simulink model "VariableCylinderTest"  (R2017b)
settings: Solver=ode15s  StartTime=0.0  StopTime=5  RelTol=1e-3  EnableMultiTasking=on
undefined symbols (not defined in the file): spring1kd, spring1ks, teth_length, teth_numLinks, teth_radius, X, Y, Z
libraries: sm_lib x16, nesl_utility x11, SimMainLibrary x5, vrlib x2, simulink x1, powerlib_meascontrol x1
settings Model: Creator=Aaron  LastModifiedBy=Aaron
settings DataIOCC: LimitDataPoints=on
settings OptimizationCC: LifeSpan=inf
settings DebuggingCC: AllowSymbolicDim=off  SFUnexpectedBacktrackingDiag=warning  SFNoUnconditionalDefaultTransitionDiag=warning  SFExecutionAtInitializationDiag=none
settings CodeAppCC: StateflowObjectComments=on
settings GRTTargetCC: TargetLangStandard=C89/C90 (ANSI)  GeneratePreprocessorConditionals=Disable all
settings ConfigComp: CovMetricSettings=dw  CovHtmlReporting=on  CovSaveCumulativeToWorkspaceVar=on  CovSaveSingleToWorkspaceVar=on  CovExternalEMLEnable=off  CovSFcnEnable=off
settings SimscapeCC: SimscapeNominalValues="[{\"value\":\"10\",\"unit\":\"V\"},{\"value\":\"1\",\"unit\":\"A\"},{\"value\":\"10\",\"unit\":\"N*m\"},{\"value\":\"10\",\"unit\":\"bar\"},{\"value\":\"100\",\"unit\":\"kJ/kg\"},{\"value\":\"1\",\"unit\":\"kW\"},{\"value\":\"300\",\"unit\":\"K\"},{\"value\":\"100\",\"unit\":\"cm^3/s\"},{\"value\":\"1\",\"unit\":\"kN\"},{\"value\":\"1\",\"unit\":\"g/cm^3\"},{\"value\":\"1\",\"unit\":\"l\"},{\"value\":\"1\",\"unit\":\"cm^2\"},{\"value\":\"60\",\"unit\":\"Hz\"}]"  SimscapeLogType=all  SimscapeLogDataHistory=10000
settings ConfigurationSet: Description=SimMechanics 2G
settings ExplorerConfigSet: InternalSimMechanicsExplorerSettings="<ExplorerConfiguration><canonicalview>default</canonicalview><AnimationSetting><BasePlaybackSpeed>1.0</BasePlaybackSpeed><PlaybackSpeedFactor>1.0</PlaybackSpeedFactor></AnimationSetting><TilePanel><TileInfo><Tiles Columns=\"1\" Count=\"1\" Rows=\"1\"><Column Weight=\"1\"/><Row Weight=\"1\"/><Tile Height=\"1\" Width=\"1\" X=\"0\" Y=\"0\"/></Tiles></TileInfo><SceneInfo><SceneViewer><BGColor><R>1</R><G>1</G><B>1</B></BGColor><Camera><DoPerspective>on</DoPerspective><Position><X>1.5</X><Y>0.241749665669615088</Y><Z>0.970338651785359607</Z></Position><Center><X>0.926423563648953952</X><Y>0.0437199328301693946</Y><Z>0.175483761522758019</Z></Center><Up><X>0.81915204428899191</X><Y>-0.138661911723834602</Y><Z>-0.556563385944725209</Z></Up><ViewLimDist>1</ViewLimDist><YLim>0.466307658154998583</YLim><XLim>1.37343348832790579</XLim></Camera></SceneViewer></SceneInfo></TilePanel><MechEditorPanel><Cameras><Camera><Id>Camera1</Id><Value><Name>Camera1</Name><NativeCamera><PositionTrackingFeature>Camera_Frame.F</PositionTrackingFeature><CenterTrackingFeature>Camera_Frame.F</CenterTrackingFeature><UpVectorTrackingFeature>Camera_Frame.F</UpVectorTrackingFeature><CenterTrackingOrigin>off</CenterTrackingOrigin><CenterTrackingDirection>-Y</CenterTrackingDirection><UpVectorTrackingDirection>+X</UpVectorTrackingDirection></NativeCamera></Value></Camera></Cameras><GfxPanelCameraMap><MapElement CameraMLId=\"Camera1\" GfxPanelIndex=\"0\"/></GfxPanelCameraMap><VideoCreator><PlaybackSpeedRatio>1.0</PlaybackSpeedRatio><FrameRate>30</FrameRate><VideoFormat>Motion JPEG AVI</VideoFormat><FrameSize>auto</FrameSize></VideoCreator></MechEditorPanel></ExplorerConfiguration>"

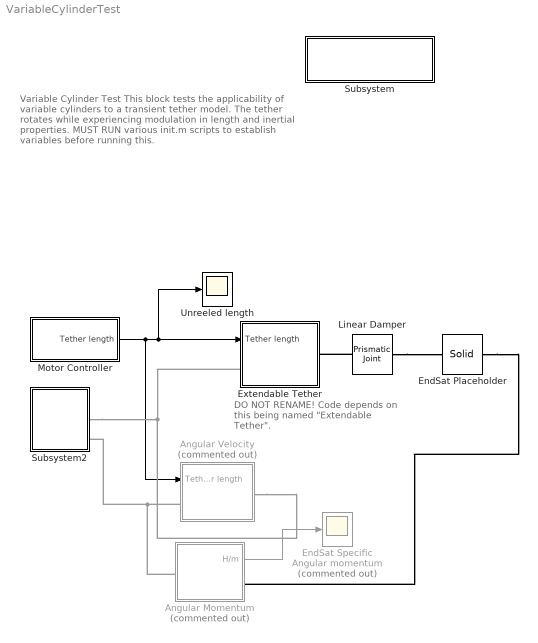
== system VariableCylinderTest ==
  note: DO NOT RENAME! Code depends on this being named "Extendable Tether".
  note: Variable Cylinder Test
      | This block tests the applicability of variable cylinders to a transient tether model. The tether rotates while experiencing modulation in length and inertial properties.
      | MUST RUN various init.m scripts to establish variables before running this.
  Angular Momentum : Subsystem  Commented=on
  Angular Velocity : Subsystem  Commented=on
  EndSat Placeholder : sm_lib/Body Elements/Solid  InertiaType=Custom  Mass=1  MassUnits=kg  CenterOfMass=[0 0 0]  CenterOfMassUnits=m  MomentsOfInertia=[.01 .01 .01]  MomentsOfInertiaUnits=kg*m^2  ProductsOfInertia=[0 0 0]  ProductsOfInertiaUnits=kg*m^2  DensityBased=off  Density=100000  DensityUnits=kg/m^3  DoExposeReferenceFrame=on  SerializedFrames=<Frames><Frame><Id>Frame1</Id><Value><Name>F1</Name><Origin><Source>GeometricFeature</Source><FeatureName>-z surface</FeatureName></Origin><PrimaryAxis><DefinedDirection>+Z</DefinedDirection><Source>ReferenceFrame</Source><SourceDirection>+Z</SourceDirection><FeatureName></FeatureName></PrimaryAxis><SecondaryAxis><DefinedDirection>+X</DefinedDirection><Source>ReferenceFrame</Source><SourceDirection>+X</SourceDirection><FeatureName></FeatureName></SecondaryAxis></Value></Frame></Frames>  GraphicType=FromGeometry  MarkerShape=Sphere  MarkerSize=10  GraphicVisPropType=SimpleVisualProperties  GraphicDiffuseColor=[0.5 0.5 0.5]  GraphicSpecularColor=[0.5 0.5 0.5 1.0]  GraphicAmbientColor=[0.15 0.15 0.15 1.0]  GraphicEmissiveColor=[0.0 0.0 0.0 1.0]  GraphicShininess=75  GraphicOpacity=1.0  GeometryShape=Brick  RectangleSize=[1 1]  RectangleSizeUnits=m  BrickDimensions=[.1 0.1 .1]  BrickDimensionUnits=m  CylinderRadius=.1  CylinderRadiusUnits=m  CylinderLength=1  CylinderLengthUnits=m  SphereRadius=1  SphereRadiusUnits=m  EllipsoidRadii=[1 1 1]  EllipsoidRadiiUnits=m  ExtrusionCrossSection=[1 1; -1 1; -1 -1; 1 -1]  ExtrusionCrossSectionUnits=m  ExtrusionLength=1  ExtrusionLengthUnits=m  PolygonNumSides=3  PolygonOuterRadius=1  PolygonOuterRadiusUnits=m  ExtGeomFileType=STEP  ExtGeomFileUnits=m  RevolutionCrossSection=[1 1; 1 -1; 2 -1; 2 1]  RevolutionCrossSectionUnits=m  RevolutionExtent=Full  RevolutionAngle=180  RevolutionAngleUnits=deg
  EndSat Specific Angular momentum : Scope  Commented=on
  Extendable Tether : Subsystem
  Linear Damper : sm_lib/Joints/Prismatic Joint  SenseConstraintForce=off  SenseConstraintForceX=off  SenseConstraintForceY=off  SenseConstraintForceZ=off  SenseConstraintTorque=off  SenseConstraintTorqueX=off  SenseConstraintTorqueY=off  SenseConstraintTorqueZ=off  SenseTotalForce=off  SenseTotalForceX=off  SenseTotalForceY=off  SenseTotalForceZ=off  SenseTotalTorque=off  SenseTotalTorqueX=off  SenseTotalTorqueY=off  SenseTotalTorqueZ=off  CompositeWrenchDir=FollowerOnBase  CompositeWrenchFrame=BaseFrame  EquilibriumPosition=0  EquilibriumPositionUnits=m  SpringStiffness=500  SpringStiffnessUnits=N/m  DampingCoefficient=50  DampingCoefficientUnits=N/(m/s)  TorqueActuationMode=NoTorque  MotionActuationMode=ComputedMotion  SensePosition=off  SenseVelocity=off  SenseAcceleration=off  SenseTorqueForce=off  PositionTargetSpecify=off  PositionTargetPriority=High  PositionTargetValue=0  PositionTargetValueUnits=m  VelocityTargetSpecify=off  VelocityTargetPriority=High  VelocityTargetValue=0  VelocityTargetValueUnits=m/s
  Motor Controller : Subsystem
  Subsystem : Subsystem
      settings: OpenFcn=open_system('sm_lib')
      mask Display: disp(sprintf('Open Simscape Multibody\nLibrary'));
  Subsystem2 : Subsystem
  Unreeled length : Scope
  wires:
  Angular Momentum/1(H/m) -> EndSat Specific Angular momentum/1
  Motor Controller/1(Tether length) -> Extendable Tether/1(Tether length), Unreeled length/1, Angular Velocity/1(Tether length)
  connections:
  EndSat Placeholder/RConn1 -- Angular Momentum/RConn1
  Linear Damper/RConn1 -- Extendable Tether/RConn1
  Linear Damper/LConn1 -- EndSat Placeholder/LConn1
  Angular Velocity/RConn1 -- Subsystem2/RConn2 -- Extendable Tether/LConn1
  Angular Velocity/LConn1 -- Subsystem2/RConn3 -- Angular Momentum/LConn1

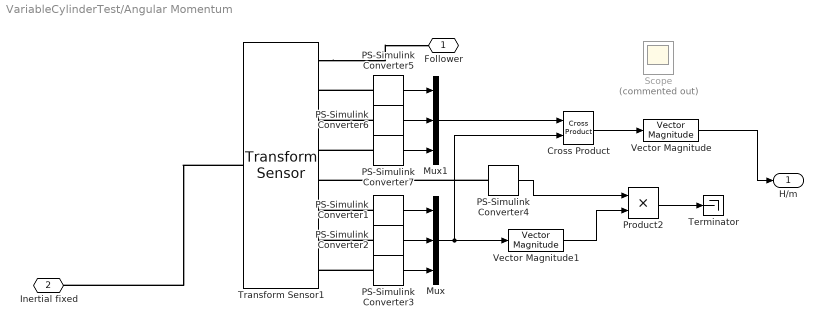
== system VariableCylinderTest/Angular Momentum ==
  Cross Product : vrlib/Utilities/Cross Product
      settings: SourceProductBaseCode=VR
  Mux : Mux  Inputs=3
  Mux1 : Mux  Inputs=3
  PS-Simulink Converter1 : nesl_utility/PS-Simulink Converter  PhysicalDomain=network_engine_domain  SubClassName=ps_output  LeftPortType=input  RightPortType=output  PseudoPeriodic=off  Frequencies=[]  Unit=m/s  AffineConversion=off
  PS-Simulink Converter2 : nesl_utility/PS-Simulink Converter  PhysicalDomain=network_engine_domain  SubClassName=ps_output  LeftPortType=input  RightPortType=output  PseudoPeriodic=off  Frequencies=[]  Unit=m/s  AffineConversion=off
  PS-Simulink Converter3 : nesl_utility/PS-Simulink Converter  PhysicalDomain=network_engine_domain  SubClassName=ps_output  LeftPortType=input  RightPortType=output  PseudoPeriodic=off  Frequencies=[]  Unit=m/s  AffineConversion=off
  PS-Simulink Converter{4..7} (4 alike) : nesl_utility/PS-Simulink Converter  PhysicalDomain=network_engine_domain  SubClassName=ps_output  LeftPortType=input  RightPortType=output  PseudoPeriodic=off  Frequencies=[]  Unit=m  AffineConversion=off
  Product2 : Product
  Scope : Scope  Commented=on  NumInputPorts=2
  Terminator : Terminator
  Transform Sensor1 : sm_lib/Frames and Transforms/Transform Sensor  MeasurementFrame=Base  SenseAngle=off  SenseAxis=off  SenseAngle1=off  SenseAngle2=off  SenseAngle3=off  SenseQ=off  SenseR=off  SenseOmegaX=off  SenseOmegaY=off  SenseOmegaZ=off  SenseOmega1=off  SenseOmega2=off  SenseOmega3=off  SenseQDot=off  SenseRDot=off  SenseAlphaX=off  SenseAlphaY=off  SenseAlphaZ=off  SenseAlpha1=off  SenseAlpha2=off  SenseAlpha3=off  SenseQDDot=off  SenseRDDot=off  SenseX=on  SenseY=on  SenseZ=on  SenseRad=off  SenseAzim=off  SenseDist=on  SenseInc=off  SenseXDot=on  SenseYDot=on  SenseZDot=on  SenseRadDot=off  SenseAzimDot=off  SenseDistDot=off  SenseIncDot=off  SenseXDDot=off  SenseYDDot=off  SenseZDDot=off  SenseRadDDot=off  SenseAzimDDot=off  SenseDistDDot=off  SenseIncDDot=off
  Vector Magnitude : SimMainLibrary/Vector Magnitude
  Vector Magnitude1 : SimMainLibrary/Vector Magnitude
  Follower : PMIOPort  Port=1  Side=Right
  Inertial fixed : PMIOPort  Port=2  Side=Left
  H/m : Outport
  wires:
  PS-Simulink Converter2/1 -> Mux/2
  PS-Simulink Converter3/1 -> Mux/3
  PS-Simulink Converter4/1 -> Product2/1
  Mux/1 -> Vector Magnitude1/1, Cross Product/2
  PS-Simulink Converter1/1 -> Mux/1
  Vector Magnitude1/1 -> Product2/2
  PS-Simulink Converter7/1 -> Mux1/3
  PS-Simulink Converter5/1 -> Mux1/1
  PS-Simulink Converter6/1 -> Mux1/2
  Mux1/1 -> Cross Product/1
  Product2/1 -> Terminator/1
  Vector Magnitude/1 -> H/m/1
  Cross Product/1 -> Vector Magnitude/1
  connections:
  PS-Simulink Converter3/LConn1 -- Transform Sensor1/RConn8
  Transform Sensor1/LConn1 -- Inertial fixed/RConn1
  Transform Sensor1/RConn1 -- Follower/RConn1
  PS-Simulink Converter2/LConn1 -- Transform Sensor1/RConn7
  PS-Simulink Converter4/LConn1 -- Transform Sensor1/RConn5
  PS-Simulink Converter1/LConn1 -- Transform Sensor1/RConn6
  PS-Simulink Converter5/LConn1 -- Transform Sensor1/RConn2
  PS-Simulink Converter6/LConn1 -- Transform Sensor1/RConn3
  PS-Simulink Converter7/LConn1 -- Transform Sensor1/RConn4

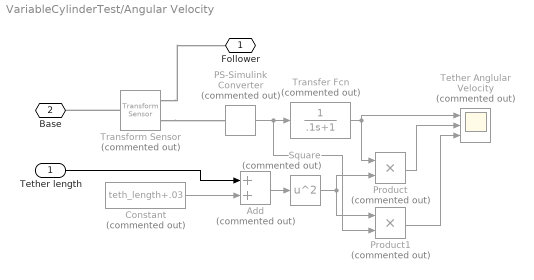
== system VariableCylinderTest/Angular Velocity ==
  Tether length : Inport
  Add : Sum  Commented=on
  Constant : Constant  Commented=on  Value=teth_length+.03
  PS-Simulink Converter : nesl_utility/PS-Simulink Converter  Commented=on  PhysicalDomain=network_engine_domain  SubClassName=ps_output  LeftPortType=input  RightPortType=output  PseudoPeriodic=off  Frequencies=[]  Unit=rad/s  AffineConversion=off
  Product : Product  Commented=on
  Product1 : Product  Commented=on
  Square : Math  Commented=on  Operator=square  RndMeth=Zero  SaturateOnIntegerOverflow=on
  Tether Anglular Velocity : Scope  Commented=on  NumInputPorts=3
  Transfer Fcn : TransferFcn  Commented=on  Denominator=[.1 1]
  Transform Sensor : sm_lib/Frames and Transforms/Transform Sensor  Commented=on  MeasurementFrame=Base  SenseAngle=off  SenseAxis=off  SenseAngle1=off  SenseAngle2=off  SenseAngle3=off  SenseQ=off  SenseR=off  SenseOmegaX=on  SenseOmegaY=off  SenseOmegaZ=off  SenseOmega1=off  SenseOmega2=off  SenseOmega3=off  SenseQDot=off  SenseRDot=off  SenseAlphaX=off  SenseAlphaY=off  SenseAlphaZ=off  SenseAlpha1=off  SenseAlpha2=off  SenseAlpha3=off  SenseQDDot=off  SenseRDDot=off  SenseX=off  SenseY=off  SenseZ=off  SenseRad=off  SenseAzim=off  SenseDist=off  SenseInc=off  SenseXDot=off  SenseYDot=off  SenseZDot=off  SenseRadDot=off  SenseAzimDot=off  SenseDistDot=off  SenseIncDot=off  SenseXDDot=off  SenseYDDot=off  SenseZDDot=off  SenseRadDDot=off  SenseAzimDDot=off  SenseDistDDot=off  SenseIncDDot=off
  Follower : PMIOPort  Port=1  Side=Right
  Base : PMIOPort  Port=2  Side=Left
  wires:
  Product1/1 -> Tether Anglular Velocity/3
  Tether length/1 -> Add/1
  Product/1 -> Tether Anglular Velocity/2
  Transfer Fcn/1 -> Product/1, Tether Anglular Velocity/1
  Add/1 -> Square/1
  Constant/1 -> Add/2
  Square/1 -> Product1/1, Product/2
  PS-Simulink Converter/1 -> Product1/2, Transfer Fcn/1
  connections:
  Transform Sensor/RConn1 -- Follower/RConn1
  Transform Sensor/LConn1 -- Base/RConn1
  Transform Sensor/RConn2 -- PS-Simulink Converter/LConn1

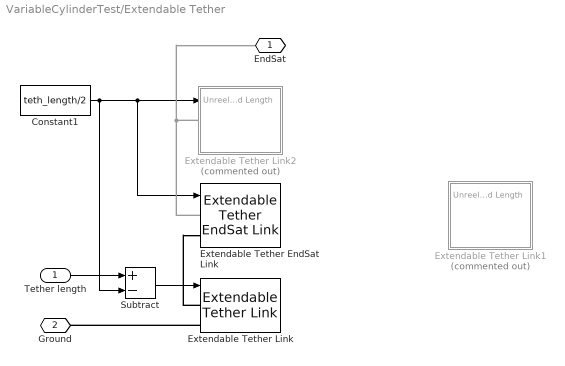
== system VariableCylinderTest/Extendable Tether ==
  Tether length : Inport
  Constant1 : Constant  Value=teth_length/2
  Extendable Tether EndSat Link : SimMainLibrary/Extendable Tether EndSat Link
  Extendable Tether Link : SimMainLibrary/Extendable Tether Link
  Extendable Tether Link1 : Subsystem  Commented=on
  Extendable Tether Link2 : Subsystem  Commented=on
  Subtract : Sum  Inputs=+-
  EndSat : PMIOPort  Port=1  Side=Right
  Ground : PMIOPort  Port=2  Side=Left
  wires:
  Constant1/1 -> Subtract/2, Extendable Tether EndSat Link/1, Extendable Tether Link2/1(Unreeled Length)
  Tether length/1 -> Subtract/1
  Subtract/1 -> Extendable Tether Link/1
  connections:
  Extendable Tether Link/LConn1 -- Extendable Tether EndSat Link/LConn2
  Extendable Tether Link/LConn2 -- Ground/RConn1
  Extendable Tether Link2/LConn1 -- Extendable Tether EndSat Link/LConn1 -- EndSat/RConn1

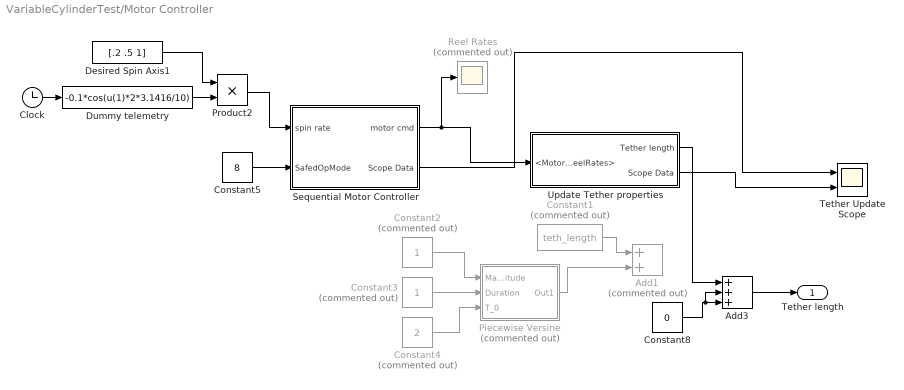
== system VariableCylinderTest/Motor Controller ==
  Add1 : Sum  Commented=on
  Add3 : Sum  Inputs=+++
  Clock : Clock
  Constant1 : Constant  Commented=on  Value=teth_length
  Constant2 : Constant  Commented=on
  Constant3 : Constant  Commented=on
  Constant4 : Constant  Commented=on  Value=2
  Constant5 : Constant  Value=8
  Constant8 : Constant  Value=0
  Desired Spin Axis1 : Constant  Value=[.2 .5 1]
  Dummy telemetry : Fcn  Expr=-0.1*cos(u(1)*2*3.1416/10)
  Piecewise Versine : Subsystem  Commented=on
  Product2 : Product
  "Reel Rates " : Scope  Commented=on
  "Sequential Motor Controller " : Subsystem  AncestorBlock=SimMainLibrary/Sequential Motor Controller
  Tether Update Scope : Scope  NumInputPorts=2
  Update Tether properties : Subsystem  AncestorBlock=SimMainLibrary/Update Tether properties
  Tether length : Outport
  wires:
  Product2/1 -> "Sequential Motor Controller "/1(spin rate)
  Constant5/1 -> "Sequential Motor Controller "/2(SafedOpMode)
  Update Tether properties/2(Scope Data) -> Tether Update Scope/2
  Constant2/1 -> Piecewise Versine/1(Magnitude)
  Piecewise Versine/1(Out1) -> Add1/2
  "Sequential Motor Controller "/1(motor cmd) -> Update Tether properties/1(<MotorReelRates>), "Reel Rates "/1
  Constant1/1 -> Add1/1
  Constant4/1 -> Piecewise Versine/3(T_0)
  Constant3/1 -> Piecewise Versine/2(Duration)
  Constant8/1 -> Add3/2, Add3/3
  Add3/1 -> Tether length/1
  Update Tether properties/1(Tether length) -> Add3/1
  Dummy telemetry/1 -> Product2/2
  Clock/1 -> Dummy telemetry/1
  Desired Spin Axis1/1 -> Product2/1
  "Sequential Motor Controller "/2(Scope Data) -> Tether Update Scope/1

== system VariableCylinderTest/Subsystem ==

== system VariableCylinderTest/Subsystem2 ==
  Camera Frame : sm_lib/Frames and Transforms/Rigid Transform  TranslationMethod=Cartesian  TranslationStandardOffset=0  TranslationLengthUnit=m  TranslationStandardAxis=+Z  TranslationCartesianOffset=[1.5 1 0]  TranslationROffset=0  TranslationROffsetUnits=m  TranslationZOffset=0  TranslationZOffsetUnits=m  TranslationThetaOffset=0  TranslationThetaOffsetUnits=deg  RotationMethod=StandardAxis  RotationAngleUnits=deg  RotationStandardAxis=+Z  RotationAngle=-35  RotationArbitraryAxis=[0 0 1]  FollAlignAxisA=+X  BaseAlignAxisA=+Y  FollAlignAxisB=+Y  BaseAlignAxisB=+Z  RotationSequenceAxes=FollowerAxes  RotationSequence=XYX  RotationSequenceAngles=[0 0 0]  RotationSequenceAnglesUnits=deg  RotationMatrix=[1 0 0; 0 1 0; 0 0 1]
  Mechanism Configuration : sm_lib/Utilities/Mechanism Configuration  UniformGravity=None  GravityVector=[0 0 -9.80665]  GravityUnits=m/s^2  LinearizationDelta=0.001
  Rigid Transform : sm_lib/Frames and Transforms/Rigid Transform  TranslationMethod=StandardAxis  TranslationStandardOffset=0  TranslationLengthUnit=m  TranslationStandardAxis=+Y  TranslationCartesianOffset=[0 0 0]  TranslationROffset=0  TranslationROffsetUnits=m  TranslationZOffset=0  TranslationZOffsetUnits=m  TranslationThetaOffset=0  TranslationThetaOffsetUnits=deg  RotationMethod=StandardAxis  RotationAngleUnits=deg  RotationStandardAxis=+X  RotationAngle=90  RotationArbitraryAxis=[0 0 1]  FollAlignAxisA=+X  BaseAlignAxisA=+Y  FollAlignAxisB=+Y  BaseAlignAxisB=+Z  RotationSequenceAxes=FollowerAxes  RotationSequence=XYX  RotationSequenceAngles=[0 0 0]  RotationSequenceAnglesUnits=deg  RotationMatrix=[1 0 0; 0 1 0; 0 0 1]
  Solver Configuration : nesl_utility/Solver Configuration  PhysicalDomain=network_engine_domain  SubClassName=solver  LeftPortType=input  RightPortType=generic  Accelerate=off  Tones=[]  Harmonics=[]  SimulateNoise=off  Profile=off  UseLocalSampling=off  EnableSwitchedLinearOptims=on  FrequencyDomain=off  UseCCode=off  RelTol=0.001  AbsTol=1e-06  MinStep=1e-09  ToWorkspace=off  RevertToSquareIcSolve=off  NumHomotopyIterations=100  PhasorMode=off  PhasorModeNumHarmonics=1  DoDC=off  ResidualTolerance=1e-09  UseLocalSolver=off  LocalSolverChoice=NE_BACKWARD_EULER_ADVANCER  LocalSolverSampleTime=0.001  DoFixedCost=off  MaxNonlinIter=3  MaxModeIter=2  LinearAlgebra=Sparse  DelaysMemoryBudget=1024  AutomaticFiltering=on  FilteringTimeConstant=0.001
  Spherical Joint : sm_lib/Joints/Spherical Joint  SenseConstraintForce=off  SenseConstraintForceX=off  SenseConstraintForceY=off  SenseConstraintForceZ=off  SenseConstraintTorque=off  SenseConstraintTorqueX=off  SenseConstraintTorqueY=off  SenseConstraintTorqueZ=off  SenseTotalForce=off  SenseTotalForceX=off  SenseTotalForceY=off  SenseTotalForceZ=off  SenseTotalTorque=off  SenseTotalTorqueX=off  SenseTotalTorqueY=off  SenseTotalTorqueZ=off  CompositeWrenchDir=FollowerOnBase  CompositeWrenchFrame=BaseFrame  DefPosRotationMethod=None  DefPosRotationAngleUnits=deg  DefPosRotationStandardAxis=+Z  DefPosRotationAngle=0.0  DefPosRotationArbitraryAxis=[0 0 1]  DefPosFollAlignAxisA=+X  DefPosBaseAlignAxisA=+Y  DefPosFollAlignAxisB=+Y  DefPosBaseAlignAxisB=+Z  DefPosRotationSequenceAxes=FollowerAxes  DefPosRotationSequence=XYX  DefPosRotationSequenceAngles=[0 0 0]  DefPosRotationSequenceAnglesUnits=deg  DefPosRotationMatrix=[1 0 0; 0 1 0; 0 0 1]  EqPosRotationMethod=None  EqPosRotationAngleUnits=deg  EqPosRotationStandardAxis=+Z  EqPosRotationAngle=0.0  EqPosRotationArbitraryAxis=[0 0 1]  EqPosFollAlignAxisA=+X  EqPosBaseAlignAxisA=+Y  EqPosFollAlignAxisB=+Y  EqPosBaseAlignAxisB=+Z  EqPosRotationSequenceAxes=FollowerAxes  EqPosRotationSequence=XYX  EqPosRotationSequenceAngles=[0 0 0]  EqPosRotationSequenceAnglesUnits=deg  EqPosRotationMatrix=[1 0 0; 0 1 0; 0 0 1]  SpringStiffness=0  SpringStiffnessUnits=N*m/deg  DampingCoefficient=0  DampingCoefficientUnits=N*m/(deg/s)  ActuateTorqueX=off  ActuateTorqueY=off  ActuateTorqueZ=off  ActuateTorque=off  TorqueActuationMode=NoTorque  MotionActuationMode=ComputedMotion  ActuationFrame=BaseFrame  SensePosition=off  SenseVelocityX=off  SenseVelocityY=off  SenseVelocityZ=off  SenseVelocity=off  SenseAccelerationX=off  SenseAccelerationY=off  SenseAccelerationZ=off  SenseAcceleration=off  SenseTorqueX=off  SenseTorqueY=off  SenseTorqueZ=off  SenseTorqueForce=off  SensingFrame=BaseFrame  PositionTargetRotationMethod=None  PositionTargetRotationAngleUnits=deg  PositionTargetRotationStandardAxis=+Z  PositionTargetRotationAngle=0.0  PositionTargetRotationArbitraryAxis=[0 0 1]  PositionTargetFollAlignAxisA=+X  PositionTargetBaseAlignAxisA=+Y  PositionTargetFollAlignAxisB=+Y  PositionTargetBaseAlignAxisB=+Z  PositionTargetRotationSequenceAxes=FollowerAxes  PositionTargetRotationSequence=XYX  PositionTargetRotationSequenceAngles=[0 0 0]  PositionTargetRotationSequenceAnglesUnits=deg  PositionTargetRotationMatrix=[1 0 0; 0 1 0; 0 0 1]  PositionTargetSpecify=off  PositionTargetPriority=High  VelocityTargetValue=[1 0 0]  VelocityTargetValueUnits=rad/s  VelocityTargetSpecify=on  VelocityTargetPriority=High  VelocityTargetInFollowerFrame=on
  World Frame : sm_lib/Frames and Transforms/World Frame
  Camera : PMIOPort  Port=1  Side=Right
  Spherical : PMIOPort  Port=2  Side=Right
  World : PMIOPort  Port=3  Side=Right
  connections:
  Camera Frame/RConn1 -- Camera/RConn1
  Camera Frame/LConn1 -- Spherical Joint/RConn1 -- Rigid Transform/LConn1
  Mechanism Configuration/RConn1 -- World/RConn1 -- World Frame/RConn1 -- Spherical Joint/LConn1 -- Solver Configuration/RConn1
  Rigid Transform/RConn1 -- Spherical/RConn1

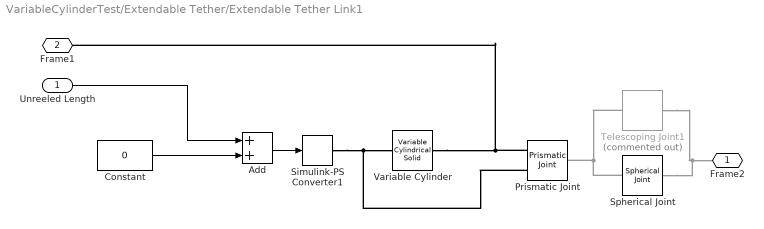
== system VariableCylinderTest/Extendable Tether/Extendable Tether Link1 ==
  Unreeled Length : Inport
  Add : Sum
  Constant : Constant  Value=0
  Prismatic Joint : sm_lib/Joints/Prismatic Joint  SenseConstraintForce=off  SenseConstraintForceX=off  SenseConstraintForceY=off  SenseConstraintForceZ=off  SenseConstraintTorque=off  SenseConstraintTorqueX=off  SenseConstraintTorqueY=off  SenseConstraintTorqueZ=off  SenseTotalForce=off  SenseTotalForceX=off  SenseTotalForceY=off  SenseTotalForceZ=off  SenseTotalTorque=off  SenseTotalTorqueX=off  SenseTotalTorqueY=off  SenseTotalTorqueZ=off  CompositeWrenchDir=FollowerOnBase  CompositeWrenchFrame=BaseFrame  EquilibriumPosition=teth_length*3  EquilibriumPositionUnits=m  SpringStiffness=spring1ks  SpringStiffnessUnits=N/m  DampingCoefficient=spring1kd  DampingCoefficientUnits=N/(m/s)  TorqueActuationMode=ComputedTorque  MotionActuationMode=InputMotion  SensePosition=off  SenseVelocity=off  SenseAcceleration=off  SenseTorqueForce=off  PositionTargetSpecify=off  PositionTargetPriority=High  PositionTargetValue=teth_length  PositionTargetValueUnits=m  VelocityTargetSpecify=off  VelocityTargetPriority=High  VelocityTargetValue=0  VelocityTargetValueUnits=m/s
  Simulink-PS Converter1 : nesl_utility/Simulink-PS Converter  PhysicalDomain=network_engine_domain  SubClassName=ps_input  LeftPortType=input  RightPortType=output  PseudoPeriodic=off  Frequencies=[]  NoiseDistribution=none  NoiseParameters=[]  Unit=m  AffineConversion=off  FilteringAndDerivatives=filter  SimscapeFilterOrder=2  InputFilterTimeConstant=0.001  UdotUserProvided=0
  Spherical Joint : sm_lib/Joints/Spherical Joint  SenseConstraintForce=off  SenseConstraintForceX=off  SenseConstraintForceY=off  SenseConstraintForceZ=off  SenseConstraintTorque=off  SenseConstraintTorqueX=off  SenseConstraintTorqueY=off  SenseConstraintTorqueZ=off  SenseTotalForce=off  SenseTotalForceX=off  SenseTotalForceY=off  SenseTotalForceZ=off  SenseTotalTorque=off  SenseTotalTorqueX=off  SenseTotalTorqueY=off  SenseTotalTorqueZ=off  CompositeWrenchDir=FollowerOnBase  CompositeWrenchFrame=BaseFrame  DefPosRotationMethod=None  DefPosRotationAngleUnits=deg  DefPosRotationStandardAxis=+Z  DefPosRotationAngle=0.0  DefPosRotationArbitraryAxis=[0 0 1]  DefPosFollAlignAxisA=+X  DefPosBaseAlignAxisA=+Y  DefPosFollAlignAxisB=+Y  DefPosBaseAlignAxisB=+Z  DefPosRotationSequenceAxes=FollowerAxes  DefPosRotationSequence=XYX  DefPosRotationSequenceAngles=[0 0 0]  DefPosRotationSequenceAnglesUnits=deg  DefPosRotationMatrix=[1 0 0; 0 1 0; 0 0 1]  EqPosRotationMethod=None  EqPosRotationAngleUnits=deg  EqPosRotationStandardAxis=+Z  EqPosRotationAngle=0.0  EqPosRotationArbitraryAxis=[0 0 1]  EqPosFollAlignAxisA=+X  EqPosBaseAlignAxisA=+Y  EqPosFollAlignAxisB=+Y  EqPosBaseAlignAxisB=+Z  EqPosRotationSequenceAxes=FollowerAxes  EqPosRotationSequence=XYX  EqPosRotationSequenceAngles=[0 0 0]  EqPosRotationSequenceAnglesUnits=deg  EqPosRotationMatrix=[1 0 0; 0 1 0; 0 0 1]  SpringStiffness=0  SpringStiffnessUnits=N*m/deg  DampingCoefficient=0  DampingCoefficientUnits=N*m/(deg/s)  ActuateTorqueX=off  ActuateTorqueY=off  ActuateTorqueZ=off  ActuateTorque=off  TorqueActuationMode=NoTorque  MotionActuationMode=ComputedMotion  ActuationFrame=BaseFrame  SensePosition=off  SenseVelocityX=off  SenseVelocityY=off  SenseVelocityZ=off  SenseVelocity=off  SenseAccelerationX=off  SenseAccelerationY=off  SenseAccelerationZ=off  SenseAcceleration=off  SenseTorqueX=off  SenseTorqueY=off  SenseTorqueZ=off  SenseTorqueForce=off  SensingFrame=BaseFrame  PositionTargetRotationMethod=None  PositionTargetRotationAngleUnits=deg  PositionTargetRotationStandardAxis=+Z  PositionTargetRotationAngle=0.0  PositionTargetRotationArbitraryAxis=[0 0 1]  PositionTargetFollAlignAxisA=+X  PositionTargetBaseAlignAxisA=+Y  PositionTargetFollAlignAxisB=+Y  PositionTargetBaseAlignAxisB=+Z  PositionTargetRotationSequenceAxes=FollowerAxes  PositionTargetRotationSequence=XYX  PositionTargetRotationSequenceAngles=[0 0 0]  PositionTargetRotationSequenceAnglesUnits=deg  PositionTargetRotationMatrix=[1 0 0; 0 1 0; 0 0 1]  PositionTargetSpecify=off  PositionTargetPriority=High  VelocityTargetValue=[0 0 0]  VelocityTargetValueUnits=deg/s  VelocityTargetSpecify=off  VelocityTargetPriority=High  VelocityTargetInFollowerFrame=on
  Telescoping Joint1 : sm_lib/Joints/Telescoping Joint  Commented=on  SenseConstraintForce=off  SenseConstraintForceX=off  SenseConstraintForceY=off  SenseConstraintForceZ=off  SenseConstraintTorque=off  SenseConstraintTorqueX=off  SenseConstraintTorqueY=off  SenseConstraintTorqueZ=off  SenseTotalForce=off  SenseTotalForceX=off  SenseTotalForceY=off  SenseTotalForceZ=off  SenseTotalTorque=off  SenseTotalTorqueX=off  SenseTotalTorqueY=off  SenseTotalTorqueZ=off  CompositeWrenchDir=FollowerOnBase  CompositeWrenchFrame=BaseFrame  SphDefPosRotationMethod=None  SphDefPosRotationAngleUnits=deg  SphDefPosRotationStandardAxis=+Z  SphDefPosRotationAngle=0.0  SphDefPosRotationArbitraryAxis=[0 0 1]  SphDefPosFollAlignAxisA=+X  SphDefPosBaseAlignAxisA=+Y  SphDefPosFollAlignAxisB=+Y  SphDefPosBaseAlignAxisB=+Z  SphDefPosRotationSequenceAxes=FollowerAxes  SphDefPosRotationSequence=XYX  SphDefPosRotationSequenceAngles=[0 0 0]  SphDefPosRotationSequenceAnglesUnits=deg  SphDefPosRotationMatrix=[1 0 0; 0 1 0; 0 0 1]  SphEqPosRotationMethod=None  SphEqPosRotationAngleUnits=deg  SphEqPosRotationStandardAxis=+Z  SphEqPosRotationAngle=0.0  SphEqPosRotationArbitraryAxis=[0 0 1]  SphEqPosFollAlignAxisA=+X  SphEqPosBaseAlignAxisA=+Y  SphEqPosFollAlignAxisB=+Y  SphEqPosBaseAlignAxisB=+Z  SphEqPosRotationSequenceAxes=FollowerAxes  SphEqPosRotationSequence=XYX  SphEqPosRotationSequenceAngles=[0 0 0]  SphEqPosRotationSequenceAnglesUnits=deg  SphEqPosRotationMatrix=[1 0 0; 0 1 0; 0 0 1]  SphSpringStiffness=0  SphSpringStiffnessUnits=N*m/deg  SphDampingCoefficient=0  SphDampingCoefficientUnits=N*m/(deg/s)  SphActuateTorqueX=off  SphActuateTorqueY=off  SphActuateTorqueZ=off  SphActuateTorque=off  SphTorqueActuationMode=NoTorque  SphMotionActuationMode=ComputedMotion  SphActuationFrame=BaseFrame  SphSensePosition=off  SphSenseVelocityX=off  SphSenseVelocityY=off  SphSenseVelocityZ=off  SphSenseVelocity=off  SphSenseAccelerationX=off  SphSenseAccelerationY=off  SphSenseAccelerationZ=off  SphSenseAcceleration=off  SphSenseTorqueX=off  SphSenseTorqueY=off  SphSenseTorqueZ=off  SphSenseTorqueForce=off  SphSensingFrame=BaseFrame  SphPositionTargetRotationMethod=None  SphPositionTargetRotationAngleUnits=deg  SphPositionTargetRotationStandardAxis=+Z  SphPositionTargetRotationAngle=0.0  SphPositionTargetRotationArbitraryAxis=[0 0 1]  SphPositionTargetFollAlignAxisA=+X  SphPositionTargetBaseAlignAxisA=+Y  SphPositionTargetFollAlignAxisB=+Y  SphPositionTargetBaseAlignAxisB=+Z  SphPositionTargetRotationSequenceAxes=FollowerAxes  SphPositionTargetRotationSequence=XYX  SphPositionTargetRotationSequenceAngles=[0 0 0]  SphPositionTargetRotationSequenceAnglesUnits=deg  SphPositionTargetRotationMatrix=[1 0 0; 0 1 0; 0 0 1]  SphPositionTargetSpecify=off  SphPositionTargetPriority=High  SphVelocityTargetValue=[0 0 0]  SphVelocityTargetValueUnits=deg/s  SphVelocityTargetSpecify=off  SphVelocityTargetPriority=High  SphVelocityTargetInFollowerFrame=on  PzEquilibriumPosition=0  PzEquilibriumPositionUnits=m  PzSpringStiffness=50  PzSpringStiffnessUnits=N/m  PzDampingCoefficient=0  PzDampingCoefficientUnits=N/(m/s)  PzTorqueActuationMode=NoTorque  PzMotionActuationMode=ComputedMotion  PzSensePosition=off  PzSenseVelocity=off  PzSenseAcceleration=off  PzSenseTorqueForce=off  PzPositionTargetSpecify=off  PzPositionTargetPriority=High  PzPositionTargetValue=0  PzPositionTargetValueUnits=m  PzVelocityTargetSpecify=off  PzVelocityTargetPriority=High  PzVelocityTargetValue=0  PzVelocityTargetValueUnits=m/s
      settings: SourceProductName=Simscape Multibody  SourceProductBaseCode=MS
  Variable Cylinder : sm_lib/Body Elements/Variable Mass/Variable Cylindrical Solid  LengthType=ProvidedByInput  Length=1  LengthUnits=m  RadiusType=Constant  Radius=teth_radius*3  RadiusUnits=m  MassType=CalculateFromGeometry  InitialMassType=Specified  InitialMass=1  InitialMassUnits=kg  Density=teth_density  DensityUnits=kg/m^3  SenseRadius=off  SenseLength=off  SenseMass=off  SenseCenterOfMass=off  SenseInertiaMatrix=off  GraphicType=FromGeometry  MarkerShape=Frame  MarkerSize=10  GraphicVisPropType=SimpleVisualProperties  GraphicDiffuseColor=[0.4 1.0 0.0]  GraphicSpecularColor=[0.5 0.5 0.5 1.0]  GraphicAmbientColor=[0.15 0.15 0.15 1.0]  GraphicEmissiveColor=[0.0 0.0 0.0 1.0]  GraphicShininess=75  GraphicOpacity=1.0
      settings: SourceProductName=Simscape Multibody  SourceProductBaseCode=MS
  Frame2 : PMIOPort  Port=1  Side=Left
  Frame1 : PMIOPort  Port=2  Side=Left
  wires:
  Unreeled Length/1 -> Add/1
  Constant/1 -> Add/2
  Add/1 -> Simulink-PS Converter1/1
  connections:
  Variable Cylinder/RConn1 -- Prismatic Joint/LConn1 -- Frame1/RConn1
  Simulink-PS Converter1/RConn1 -- Prismatic Joint/LConn2 -- Variable Cylinder/LConn1
  Telescoping Joint1/LConn1 -- Spherical Joint/LConn1 -- Prismatic Joint/RConn1
  Telescoping Joint1/RConn1 -- Spherical Joint/RConn1 -- Frame2/RConn1

== system VariableCylinderTest/Extendable Tether/Extendable Tether Link2 ==
  Unreeled Length : Inport
  Add : Sum
  Constant : Constant  Value=0
  Prismatic Joint : sm_lib/Joints/Prismatic Joint  SenseConstraintForce=off  SenseConstraintForceX=off  SenseConstraintForceY=off  SenseConstraintForceZ=off  SenseConstraintTorque=off  SenseConstraintTorqueX=off  SenseConstraintTorqueY=off  SenseConstraintTorqueZ=off  SenseTotalForce=off  SenseTotalForceX=off  SenseTotalForceY=off  SenseTotalForceZ=off  SenseTotalTorque=off  SenseTotalTorqueX=off  SenseTotalTorqueY=off  SenseTotalTorqueZ=off  CompositeWrenchDir=FollowerOnBase  CompositeWrenchFrame=BaseFrame  EquilibriumPosition=teth_length*3  EquilibriumPositionUnits=m  SpringStiffness=spring1ks  SpringStiffnessUnits=N/m  DampingCoefficient=spring1kd  DampingCoefficientUnits=N/(m/s)  TorqueActuationMode=ComputedTorque  MotionActuationMode=InputMotion  SensePosition=off  SenseVelocity=off  SenseAcceleration=off  SenseTorqueForce=off  PositionTargetSpecify=off  PositionTargetPriority=High  PositionTargetValue=teth_length  PositionTargetValueUnits=m  VelocityTargetSpecify=off  VelocityTargetPriority=High  VelocityTargetValue=0  VelocityTargetValueUnits=m/s
  Simulink-PS Converter1 : nesl_utility/Simulink-PS Converter  PhysicalDomain=network_engine_domain  SubClassName=ps_input  LeftPortType=input  RightPortType=output  PseudoPeriodic=off  Frequencies=[]  NoiseDistribution=none  NoiseParameters=[]  Unit=m  AffineConversion=off  FilteringAndDerivatives=filter  SimscapeFilterOrder=2  InputFilterTimeConstant=0.001  UdotUserProvided=0
  Telescoping Joint1 : sm_lib/Joints/Telescoping Joint  SenseConstraintForce=off  SenseConstraintForceX=off  SenseConstraintForceY=off  SenseConstraintForceZ=off  SenseConstraintTorque=off  SenseConstraintTorqueX=off  SenseConstraintTorqueY=off  SenseConstraintTorqueZ=off  SenseTotalForce=off  SenseTotalForceX=off  SenseTotalForceY=off  SenseTotalForceZ=off  SenseTotalTorque=off  SenseTotalTorqueX=off  SenseTotalTorqueY=off  SenseTotalTorqueZ=off  CompositeWrenchDir=FollowerOnBase  CompositeWrenchFrame=BaseFrame  SphDefPosRotationMethod=None  SphDefPosRotationAngleUnits=deg  SphDefPosRotationStandardAxis=+Z  SphDefPosRotationAngle=0.0  SphDefPosRotationArbitraryAxis=[0 0 1]  SphDefPosFollAlignAxisA=+X  SphDefPosBaseAlignAxisA=+Y  SphDefPosFollAlignAxisB=+Y  SphDefPosBaseAlignAxisB=+Z  SphDefPosRotationSequenceAxes=FollowerAxes  SphDefPosRotationSequence=XYX  SphDefPosRotationSequenceAngles=[0 0 0]  SphDefPosRotationSequenceAnglesUnits=deg  SphDefPosRotationMatrix=[1 0 0; 0 1 0; 0 0 1]  SphEqPosRotationMethod=None  SphEqPosRotationAngleUnits=deg  SphEqPosRotationStandardAxis=+Z  SphEqPosRotationAngle=0.0  SphEqPosRotationArbitraryAxis=[0 0 1]  SphEqPosFollAlignAxisA=+X  SphEqPosBaseAlignAxisA=+Y  SphEqPosFollAlignAxisB=+Y  SphEqPosBaseAlignAxisB=+Z  SphEqPosRotationSequenceAxes=FollowerAxes  SphEqPosRotationSequence=XYX  SphEqPosRotationSequenceAngles=[0 0 0]  SphEqPosRotationSequenceAnglesUnits=deg  SphEqPosRotationMatrix=[1 0 0; 0 1 0; 0 0 1]  SphSpringStiffness=0  SphSpringStiffnessUnits=N*m/deg  SphDampingCoefficient=0  SphDampingCoefficientUnits=N*m/(deg/s)  SphActuateTorqueX=off  SphActuateTorqueY=off  SphActuateTorqueZ=off  SphActuateTorque=off  SphTorqueActuationMode=NoTorque  SphMotionActuationMode=ComputedMotion  SphActuationFrame=BaseFrame  SphSensePosition=off  SphSenseVelocityX=off  SphSenseVelocityY=off  SphSenseVelocityZ=off  SphSenseVelocity=off  SphSenseAccelerationX=off  SphSenseAccelerationY=off  SphSenseAccelerationZ=off  SphSenseAcceleration=off  SphSenseTorqueX=off  SphSenseTorqueY=off  SphSenseTorqueZ=off  SphSenseTorqueForce=off  SphSensingFrame=BaseFrame  SphPositionTargetRotationMethod=None  SphPositionTargetRotationAngleUnits=deg  SphPositionTargetRotationStandardAxis=+Z  SphPositionTargetRotationAngle=0.0  SphPositionTargetRotationArbitraryAxis=[0 0 1]  SphPositionTargetFollAlignAxisA=+X  SphPositionTargetBaseAlignAxisA=+Y  SphPositionTargetFollAlignAxisB=+Y  SphPositionTargetBaseAlignAxisB=+Z  SphPositionTargetRotationSequenceAxes=FollowerAxes  SphPositionTargetRotationSequence=XYX  SphPositionTargetRotationSequenceAngles=[0 0 0]  SphPositionTargetRotationSequenceAnglesUnits=deg  SphPositionTargetRotationMatrix=[1 0 0; 0 1 0; 0 0 1]  SphPositionTargetSpecify=off  SphPositionTargetPriority=High  SphVelocityTargetValue=[0 0 0]  SphVelocityTargetValueUnits=deg/s  SphVelocityTargetSpecify=off  SphVelocityTargetPriority=High  SphVelocityTargetInFollowerFrame=on  PzEquilibriumPosition=0  PzEquilibriumPositionUnits=m  PzSpringStiffness=54.5455  PzSpringStiffnessUnits=N/m  PzDampingCoefficient=spring1kd*10000  PzDampingCoefficientUnits=N/(m/s)  PzTorqueActuationMode=NoTorque  PzMotionActuationMode=ComputedMotion  PzSensePosition=off  PzSenseVelocity=off  PzSenseAcceleration=off  PzSenseTorqueForce=off  PzPositionTargetSpecify=off  PzPositionTargetPriority=High  PzPositionTargetValue=0  PzPositionTargetValueUnits=m  PzVelocityTargetSpecify=off  PzVelocityTargetPriority=High  PzVelocityTargetValue=0  PzVelocityTargetValueUnits=m/s
      settings: SourceProductName=Simscape Multibody  SourceProductBaseCode=MS
  Variable Cylinder : sm_lib/Body Elements/Variable Mass/Variable Cylindrical Solid  LengthType=ProvidedByInput  Length=1  LengthUnits=m  RadiusType=Constant  Radius=teth_radius*10  RadiusUnits=m  MassType=CalculateFromGeometry  InitialMassType=Specified  InitialMass=1  InitialMassUnits=kg  Density=teth_density  DensityUnits=kg/m^3  SenseRadius=off  SenseLength=off  SenseMass=off  SenseCenterOfMass=off  SenseInertiaMatrix=off  GraphicType=FromGeometry  MarkerShape=Frame  MarkerSize=10  GraphicVisPropType=SimpleVisualProperties  GraphicDiffuseColor=[0.4 1.0 0.0]  GraphicSpecularColor=[0.5 0.5 0.5 1.0]  GraphicAmbientColor=[0.15 0.15 0.15 1.0]  GraphicEmissiveColor=[0.0 0.0 0.0 1.0]  GraphicShininess=75  GraphicOpacity=1.0
      settings: SourceProductName=Simscape Multibody  SourceProductBaseCode=MS
  Frame2 : PMIOPort  Port=1  Side=Left
  Frame1 : PMIOPort  Port=2  Side=Left
  wires:
  Unreeled Length/1 -> Add/1
  Constant/1 -> Add/2
  Add/1 -> Simulink-PS Converter1/1
  connections:
  Variable Cylinder/RConn1 -- Prismatic Joint/LConn1 -- Frame1/RConn1
  Simulink-PS Converter1/RConn1 -- Prismatic Joint/LConn2 -- Variable Cylinder/LConn1
  Telescoping Joint1/LConn1 -- Prismatic Joint/RConn1
  Telescoping Joint1/RConn1 -- Frame2/RConn1

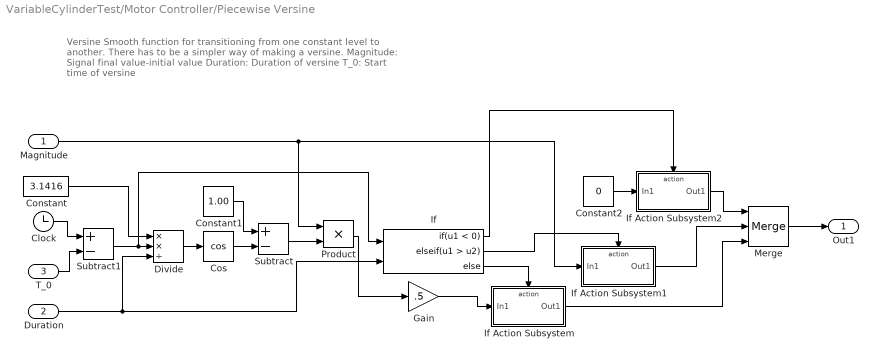
== system VariableCylinderTest/Motor Controller/Piecewise Versine ==
  note: Versine
      | Smooth function for transitioning from one constant level to another.
      | There has to be a simpler way of making a versine.
      | Magnitude: Signal final value-initial value
      | Duration: Duration of versine
      | T_0: Start time of versine
  Magnitude : Inport
  Duration : Inport  Port=2
  T_0 : Inport  Port=3
  Clock : Clock
  Constant : Constant  Value=3.1416
  Constant1 : Constant  Value=1.00
  Constant2 : Constant  Value=0
  Cos : Trigonometry  Operator=cos
  Divide : Product  Inputs=**/
  Gain : Gain  Gain=.5
  If : If  NumInputs=2  IfExpression=u1 < 0  ElseIfExpressions=u1 > u2
  If Action Subsystem : Subsystem  TreatAsAtomicUnit=on
  If Action Subsystem1 : Subsystem  TreatAsAtomicUnit=on
  If Action Subsystem2 : Subsystem  TreatAsAtomicUnit=on
  Merge : Merge  Inputs=3
  Product : Product
  Subtract : Sum  Inputs=+-
  Subtract1 : Sum  Inputs=+-
  Out1 : Outport
  wires:
  Clock/1 -> Subtract1/1
  Divide/1 -> Cos/1
  Magnitude/1 -> Product/1, If Action Subsystem1/1(In1)
  Cos/1 -> Subtract/2
  Subtract/1 -> Product/2
  Constant1/1 -> Subtract/1
  T_0/1 -> Subtract1/2
  Product/1 -> Gain/1
  Duration/1 -> If/2, Divide/3
  If/2 -> If Action Subsystem1/Action
  If/3 -> If Action Subsystem/Action
  If/1 -> If Action Subsystem2/Action
  Constant2/1 -> If Action Subsystem2/1(In1)
  If Action Subsystem2/1(Out1) -> Merge/1
  If Action Subsystem1/1(Out1) -> Merge/2
  If Action Subsystem/1(Out1) -> Merge/3
  Merge/1 -> Out1/1
  Gain/1 -> If Action Subsystem/1(In1)
  Subtract1/1 -> If/1, Divide/2
  Constant/1 -> Divide/1

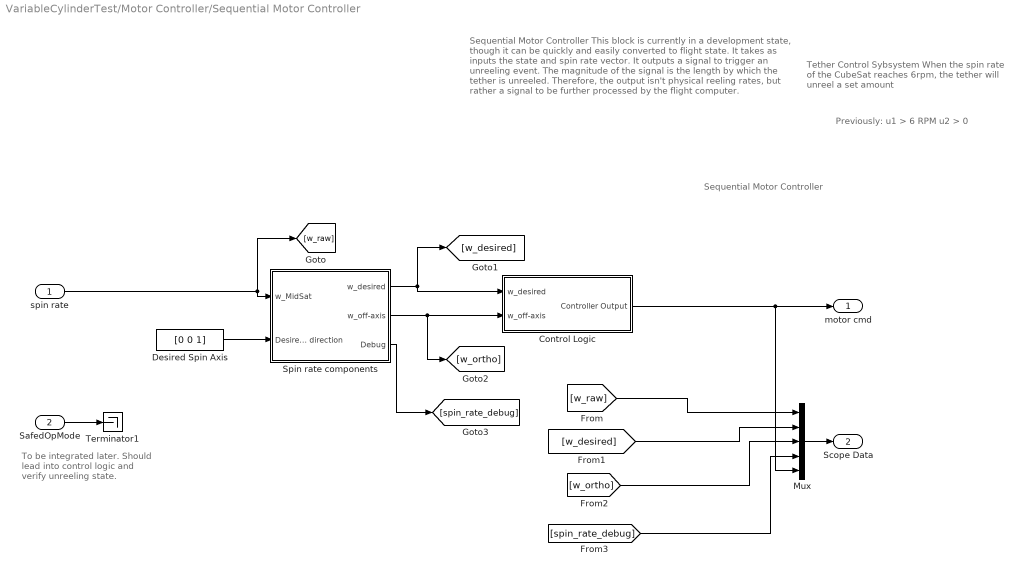
== system VariableCylinderTest/Motor Controller/Sequential Motor Controller  ==
  note: Sequential Motor Controller
  note: Tether Control Sybsystem
      | When the spin rate of the CubeSat reaches
      | 6rpm, the tether will unreel a set amount
  note: Previously:
      | u1 > 6 RPM
      | u2 > 0
  note: Sequential Motor Controller
      | This block is currently in a development state, though it can be quickly and easily converted to flight state. It takes as inputs the state and spin rate vector. It outputs a signal to trigger an unreeling event. The magnitude of the signal is the length by which the tether is unreeled. Therefore, the output isn't physical reeling rates, but rather a signal to be further processed by the flight computer.
  note: To be integrated later. Should lead into control logic and verify unreeling state.
  spin rate : Inport
  SafedOpMode : Inport  Port=2
  Control Logic : Subsystem
  Desired Spin Axis : Constant  Value=[0 0 1]
  Mux : Mux  Inputs=5
  Spin rate components : Subsystem
  Terminator1 : Terminator
  motor cmd : Outport
  Scope Data : Outport  Port=2
  wires:
  Control Logic/1(Controller Output) -> motor cmd/1, Mux/5
  spin rate/1 -> Spin rate components/1(w_MidSat), [w_raw]
  Spin rate components/3(Debug) -> [spin_rate_debug]
  [w_ortho] -> Mux/3
  [w_raw] -> Mux/1
  [w_desired] -> Mux/2
  [spin_rate_debug] -> Mux/4
  Spin rate components/2(w_off-axis) -> Control Logic/2(w_off-axis), [w_ortho]
  Desired Spin Axis/1 -> Spin rate components/2(Desired spin direction)
  Spin rate components/1(w_desired) -> Control Logic/1(w_desired), [w_desired]
  Mux/1 -> Scope Data/1
  SafedOpMode/1 -> Terminator1/1

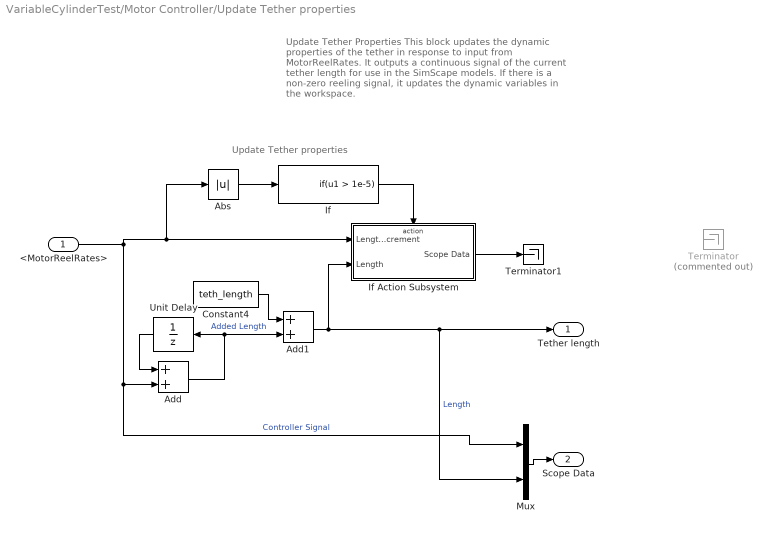
== system VariableCylinderTest/Motor Controller/Update Tether properties ==
  note: Update Tether properties
  note: Update Tether Properties
      | This block updates the dynamic properties of the tether in response to input from MotorReelRates.
      | It outputs a continuous signal of the current tether length for use in the SimScape models.
      | If there is a non-zero reeling signal, it updates the dynamic variables in the workspace.
  <MotorReelRates> : Inport
  Abs : Abs
  Add : Sum
  Add1 : Sum
  Constant4 : Constant  Value=teth_length
  If : If  IfExpression=u1 > 1e-5  ShowElse=off
  If Action Subsystem : Subsystem  TreatAsAtomicUnit=on
  Mux : Mux  Inputs=2
  Terminator : Terminator  Commented=on
  Terminator1 : Terminator
  Unit Delay : UnitDelay  SampleTime=-1
  Tether length : Outport
  Scope Data : Outport  Port=2
  wires:
  If/1 -> If Action Subsystem/Action
  <MotorReelRates>/1 -> Abs/1, If Action Subsystem/1(Length Increment), Mux/1, Add/2  "Controller Signal"
  Constant4/1 -> Add1/1
  Add/1 -> Add1/2, Unit Delay/1  "Added Length"
  Add1/1 -> Mux/2, Tether length/1, If Action Subsystem/2(Length)  "Length"
  Unit Delay/1 -> Add/1
  Abs/1 -> If/1
  Mux/1 -> Scope Data/1
  If Action Subsystem/1(Scope Data) -> Terminator1/1

== system VariableCylinderTest/Motor Controller/Piecewise Versine/If Action Subsystem ==
  In1 : Inport
  Action Port : ActionPort  ActionType=else
  Out1 : Outport
  wires:
  In1/1 -> Out1/1

== system VariableCylinderTest/Motor Controller/Piecewise Versine/If Action Subsystem1 ==
  In1 : Inport
  Action Port : ActionPort  ActionType=elseif
  Out1 : Outport
  wires:
  In1/1 -> Out1/1

== system VariableCylinderTest/Motor Controller/Piecewise Versine/If Action Subsystem2 ==
  In1 : Inport
  Action Port : ActionPort  ActionType=then
  Out1 : Outport
  wires:
  In1/1 -> Out1/1

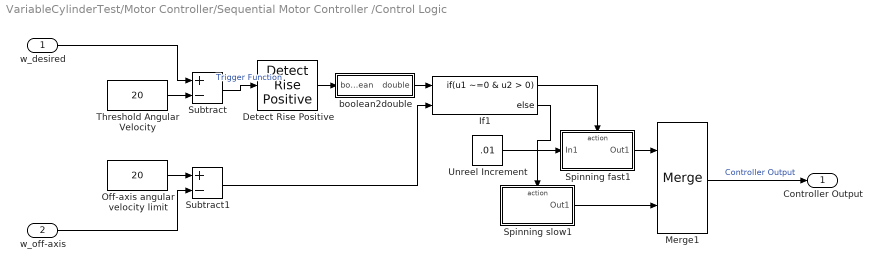
== system VariableCylinderTest/Motor Controller/Sequential Motor Controller /Control Logic ==
  w_desired : Inport
  w_off-axis : Inport  Port=2
  Detect Rise Positive : simulink/Logic and Bit Operations/Detect Rise Positive  vinit=0  OutDataTypeStr=boolean
  If1 : If  NumInputs=2  IfExpression=u1 ~=0 & u2 > 0
  Merge1 : Merge
  Off-axis angular velocity limit : Constant  Value=20
  Spinning fast1 : Subsystem  TreatAsAtomicUnit=on
  Spinning slow1 : Subsystem  TreatAsAtomicUnit=on
  Subtract : Sum  Inputs=+-
  Subtract1 : Sum  Inputs=+-
  Threshold Angular Velocity : Constant  Value=20
  Unreel Increment : Constant  Value=.01
  boolean2double : Subsystem
  Controller Output : Outport
  wires:
  Merge1/1 -> Controller Output/1  "Controller Output"
  w_off-axis/1 -> Subtract1/2
  w_desired/1 -> Subtract/1
  Off-axis angular velocity limit/1 -> Subtract1/1
  Detect Rise Positive/1 -> boolean2double/1("boolean ")
  boolean2double/1(double) -> If1/1
  Subtract1/1 -> If1/2
  Subtract/1 -> Detect Rise Positive/1  "Trigger Function"
  Spinning slow1/1(Out1) -> Merge1/2
  Threshold Angular Velocity/1 -> Subtract/2
  Unreel Increment/1 -> Spinning fast1/1(In1)
  Spinning fast1/1(Out1) -> Merge1/1
  If1/1 -> Spinning fast1/Action
  If1/2 -> Spinning slow1/Action

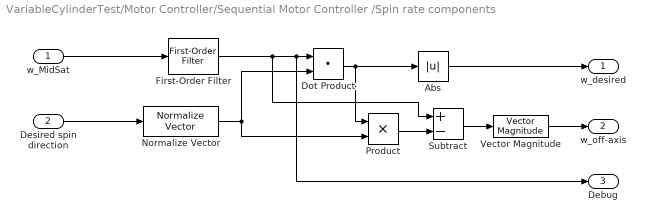
== system VariableCylinderTest/Motor Controller/Sequential Motor Controller /Spin rate components ==
  w_MidSat : Inport
  Desired spin direction : Inport  Port=2
  Abs : Abs
  Dot Product : DotProduct  InputSameDT=on  OutDataTypeStr=Inherit: Inherit via internal rule
  First-Order Filter : powerlib_meascontrol/Filters/First-Order Filter  FilterType=Lowpass  Tc=.1  Ts=0  Initialize=on  Vac_Init=[0, 0, 0]  Vdc_Init=0  PlotResponse=off  FreqRange="[0,  200,  1]"
      settings: SourceProductName=Simscape Power Systems
  Normalize Vector : vrlib/Utilities/Normalize Vector  maxzero=0
      settings: SourceProductName=Simulink 3D Animation  SourceProductBaseCode=VR
  Product : Product
  Subtract : Sum  Inputs=+-
  Vector Magnitude : SimMainLibrary/Vector Magnitude
  w_desired : Outport
  w_off-axis : Outport  Port=2
  Debug : Outport  Port=3
  wires:
  Vector Magnitude/1 -> w_off-axis/1
  Desired spin direction/1 -> Normalize Vector/1
  First-Order Filter/1 -> Subtract/1, Debug/1, Dot Product/1
  Dot Product/1 -> Product/1, Abs/1
  Abs/1 -> w_desired/1
  w_MidSat/1 -> First-Order Filter/1
  Normalize Vector/1 -> Dot Product/2, Product/2
  Product/1 -> Subtract/2
  Subtract/1 -> Vector Magnitude/1

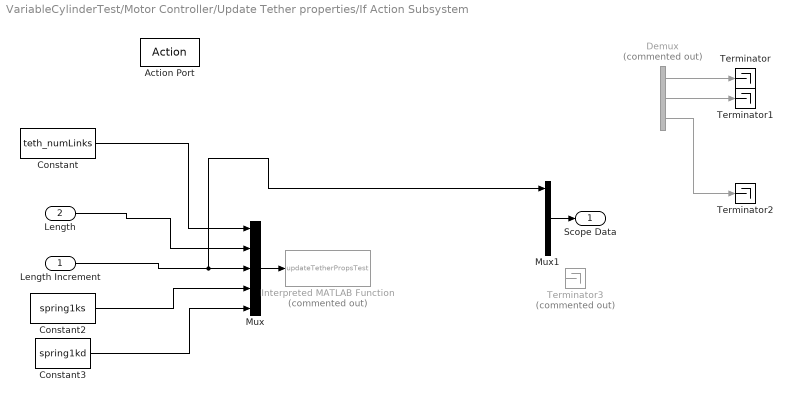
== system VariableCylinderTest/Motor Controller/Update Tether properties/If Action Subsystem ==
  Length Increment : Inport
  Length : Inport  Port=2
  Action Port : ActionPort  ActionType=then
  Constant : Constant  Value=teth_numLinks
  Constant2 : Constant  Value=spring1ks
  Constant3 : Constant  Value=spring1kd
  Demux : Demux  Commented=on  Outputs=3
  Interpreted MATLAB Function : MATLABFcn  Commented=on  MATLABFcn=updateTetherPropsTest  OutputDimensions=0  Output1D=off
  Mux : Mux  Inputs=5
  Mux1 : Mux  Inputs=5
  Terminator : Terminator
  Terminator1 : Terminator
  Terminator2 : Terminator
  Terminator3 : Terminator  Commented=on
  Scope Data : Outport
  wires:
  Demux/3 -> Terminator2/1
  Demux/2 -> Terminator1/1
  Demux/1 -> Terminator/1
  Mux/1 -> Interpreted MATLAB Function/1
  Length/1 -> Mux/2
  Constant3/1 -> Mux/5
  Constant2/1 -> Mux/4
  Length Increment/1 -> Mux1/1, Mux/3
  Constant/1 -> Mux/1
  Mux1/1 -> Scope Data/1

== system VariableCylinderTest/Motor Controller/Sequential Motor Controller /Control Logic/Spinning fast1 ==
  In1 : Inport
  Action Port : ActionPort  InitializeStates=reset  ActionType=then
  Out1 : Outport
  wires:
  In1/1 -> Out1/1

== system VariableCylinderTest/Motor Controller/Sequential Motor Controller /Control Logic/Spinning slow1 ==
  Action Port : ActionPort  ActionType=else
  Constant : Constant  Value=0
  Out1 : Outport
  wires:
  Constant/1 -> Out1/1

== system VariableCylinderTest/Motor Controller/Sequential Motor Controller /Control Logic/boolean2double ==
  "boolean " : Inport
  If : If  IfExpression=u1
  If Action Subsystem : Subsystem  TreatAsAtomicUnit=on
  Merge1 : Merge
  Spinning slow1 : Subsystem  TreatAsAtomicUnit=on
  double : Outport
  wires:
  "boolean "/1 -> If/1
  If/2 -> Spinning slow1/Action
  Spinning slow1/1(Out1) -> Merge1/2
  If Action Subsystem/1(Out1) -> Merge1/1
  Merge1/1 -> double/1
  If/1 -> If Action Subsystem/Action

== system VariableCylinderTest/Motor Controller/Sequential Motor Controller /Control Logic/boolean2double/If Action Subsystem ==
  Action Port : ActionPort  ActionType=then
  Constant : Constant
  Out1 : Outport
  wires:
  Constant/1 -> Out1/1

== system VariableCylinderTest/Motor Controller/Sequential Motor Controller /Control Logic/boolean2double/Spinning slow1 ==
  Action Port : ActionPort  ActionType=else
  Constant : Constant  Value=0
  Out1 : Outport
  wires:
  Constant/1 -> Out1/1
